simulink model "modelo_planta_CODESYS_EXPERIMENTAL"  (R2025b)
settings: Solver=FixedStepAuto  StartTime=0.0  StopTime=inf  FixedStep=Ts2  MaxStep=1e-3  RelTol=1e-3
undefined symbols (not defined in the file): ah_max, at_max, bcx, bcy, bh_eq, bhb, bhEb, bhwu, bt, bt_eq, btb, btw, g, Hc, ih, it, Jh_eq, Jt_eq, Kcy, khwu, Ki_h, Ki_t, Kp_h, Kp_t, Ktw, lambda, Lh, Lh0, lh_0, Lt, magnitude, Mc_max, Ms, Mt, rhd, rtd, tau_hm, tau_tm, Thb_Max, ThEb_Max, Thm_0, Thm_Max, titahm_0, titatm_0, Ts0, Ts1, Ts2, Ttb_Max, Ttm_0, Ttm_Max, vh_0, vlx_0, vly_0, vt_0, vt_max, Wc, whm_0, whm_rated, wtm_0, xl_0 ... (+9)
libraries: simulink x10, opcualib x9, sl3dlib x1, simulink_extras x1, dspnetwork x1
(part 1 of 2)
settings Model: SimulationMode=accelerator  Creator=Nahuel  LastModifiedBy=rodri
settings SolverCC: ZeroCrossControl=DisableAll
settings DebuggingCC: UnderSpecifiedDimensionMsg=warning
settings SFSimCC: SimTargetLang=C++  SimDLTargetLibrary=mkl-dnn
settings RTWCC: GPUComputeCapability=3.5

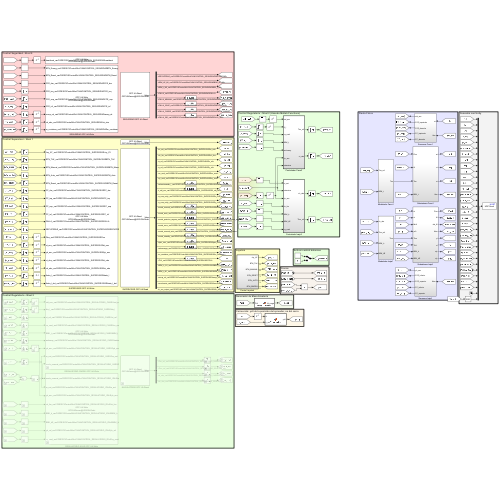
[thumbnail: Simulink's stored preview of the top-level diagram]
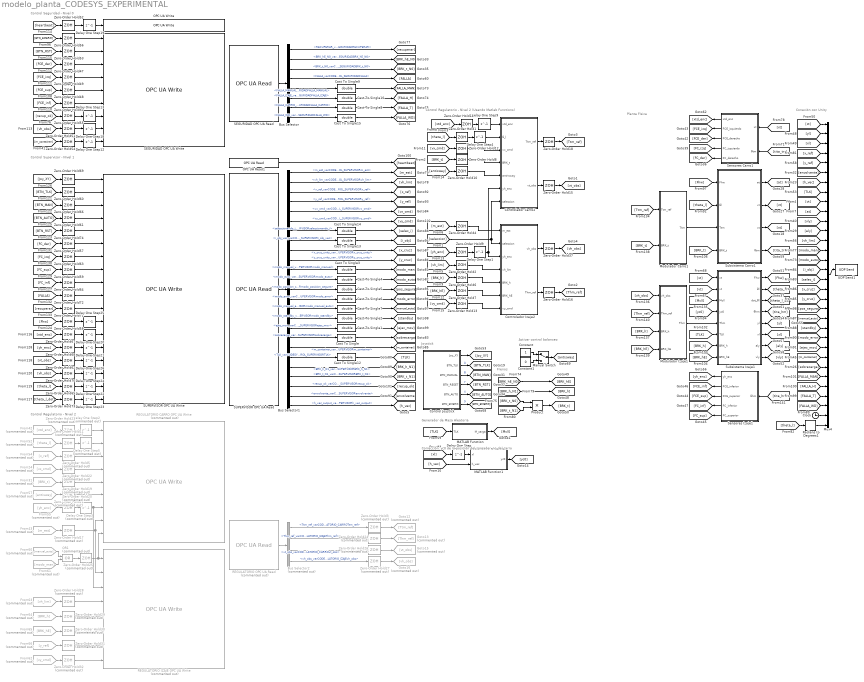
== system modelo_planta_CODESYS_EXPERIMENTAL ==
  note: Activar control balanceo
  note: Generador de Masa Aleatoria
  note: Frenos
  note: Corrección: yc0 de la posición del spreader, no del carro
  note: Joystick
  note: Conexión con Unity
  note: Control Seguridad - Nivel 0
  note: Control Supervisor - Nivel 1
  note: Control Regulatorio - Nivel 2
  note: Planta Física
  note: Control Regulatorio - Nivel 2 (Usando Matlab Functions)
  Bus Selector : BusSelector  OutputSignals=RECUPERAR_varCODESYSControlWinV3X64CONTROL_SEGURIDADRECUPERAR,BRK_hE_N0_varCODESYSControlWinV3X64CONTROL_SEGURIDADBRK_hE_N0,BRK_t_N0_varCODESYSControlWinV3X64CONTROL_SEGURIDADBRK_t_N0,FALLA_varCODESYSControlWinV3X64CONTROL_SEGURIDADFALLA,FALLA_MANUAL_varCODESYSControlWinV3X64CONTROL_SEGURIDADFALLA_MANUAL,FALLA_IZAJE_varCODESYSControlWinV3X64CONTROL_SEGURIDADFALLA_IZAJE,FALLA_CARRO_varCODESYSControlWinV3X64CONTROL_SEGURIDADFALLA_CARRO,FALLA_WD_varCODESYSControlWinV3X64CONTROL_SEGURIDADFALLA_WD
  Bus Selector1 : BusSelector  OutputSignals=m_est_varCODESYSControlWinV3X64CONTROL_SUPERVISORm_est,vh_lim_varCODESYSControlWinV3X64CONTROL_SUPERVISORvh_lim,x_ref_varCODESYSControlWinV3X64CONTROL_SUPERVISORx_ref,y_ref_varCODESYSControlWinV3X64CONTROL_SUPERVISORy_ref,vx_cmd_varCODESYSControlWinV3X64CONTROL_SUPERVISORvx_cmd,vy_cmd_varCODESYSControlWinV3X64CONTROL_SUPERVISORvy_cmd,seleccionando_i_varCODESYSControlWinV3X64CONTROL_SUPERVISORseleccionando_i,i_obj_vec_varCODESYSControlWinV3X64CONTROL_SUPERVISORi_obj_vec,x_cruz_unity_varCODESYSControlWinV3X64CONTROL_SUPERVISORx_cruz_unity,y_cruz_unity_varCODESYSControlWinV3X64CONTROL_SUPERVISORy_cruz_unity,modo_manual_varCODESYSControlWinV3X64CONTROL_SUPERVISORmodo_manual,modo_auto_varCODESYSControlWinV3X64CONTROL_SUPERVISORmodo_auto,modo_posicion_segura_varCODESYSControlWinV3X64CONTROL_SUPERVISORmodo_posicion_segura,modo_error_varCODESYSControlWinV3X64CONTROL_SUPERVISORmodo_error,modo_manual_auto_varCODESYSControlWinV3X64CONTROL_SUPERVISORmodo_manual_auto,modo_standby_varCODESYSControlWinV3X64CONTROL_SUPERVISORmodo_standby,ejec_mov_varCODESYSControlWinV3X64CONTROL_SUPERVISORejec_mov,sobrecarga_varCODESYSControlWinV3X64CONTROL_SUPERVISORsobrecarga,m_container_varCODESYSControlWinV3X64CONTROL_SUPERVISORm_container,TLK_varCODESYSControlWinV3X64CONTROL_SUPERVISORTLK,BRK_h_N1_varCODESYSControlWinV3X64CONTROL_SUPERVISORBRK_h_N1,BRK_t_N1_varCODESYSControlWinV3X64CONTROL_SUPERVISORBRK_t_N1,recup_ok_varCODESYSControlWinV3X64CONTROL_SUPERVISORrecup_ok,envolvente_varCODESYSControlWinV3X64CONTROL_SUPERVISORenvolvente,h_vec_output_varCODESYSControlWinV3X64CONTROL_SUPERVISORh_vec_output
  Bus Selector2 : BusSelector  Commented=on  OutputSignals=Ttm_ref_varCODESYSControlWinV3X64CONTROL_REGULATORIO_CARROTtm_ref,Thm_ref_varCODESYSControlWinV3X64CONTROL_REGULATORIO_IZAJEThm_ref,vt_obs_varCODESYSControlWinV3X64CONTROL_REGULATORIO_CARROvt_obs,vh_obs_varCODESYSControlWinV3X64CONTROL_REGULATORIO_IZAJEvh_obs
  Cast To Single{,1..10,12..15} (15 alike) : DataTypeConversion  OutDataTypeStr=double  SaturateOnIntegerOverflow=off  RndMeth=Floor
  Clock : Clock
  Constant : Constant
  Constant1 : Constant  Value=0
  "Control Joystick " : Subsystem  TreatAsAtomicUnit=on  SystemSampleTime=Ts2
  Controlador Carro2 : Subsystem  Priority=3  TreatAsAtomicUnit=on  SystemSampleTime=Ts2
  Controlador Izaje2 : Subsystem  Priority=3  TreatAsAtomicUnit=on  SystemSampleTime=Ts2
  Delay One Step : Delay  DelayLength=1  InitialCondition=xl_0
  Delay One Step1 : Delay  DelayLength=1  InitialCondition=yh_0
  Delay One Step{4,12..13,18..19,22..24,26} (9 alike) : Delay  DelayLength=1  InitialCondition=0
  Delay One Step2 : Delay  Commented=on  DelayLength=1  InitialCondition=xtd_0
  Delay One Step20 : Delay  DelayLength=1  InitialCondition=xt_0
  Delay One Step21 : Delay  DelayLength=1  InitialCondition=yh_0
  Delay One Step25 : Delay  DelayLength=1
  Delay One Step3 : Delay  Commented=on  DelayLength=1  InitialCondition=yh_0
  Delay One Step5 : Delay  Commented=on  DelayLength=1  InitialCondition=0
  Delay One Step9 : Delay  DelayLength=1  InitialCondition=xtd_0
  From24 : From  Commented=on  GotoTag=vx_cmd
  From31 : From  Commented=on  GotoTag=BRK_t
  From42 : From  Commented=on  GotoTag=xtd_enc
  From43 : From  Commented=on  GotoTag=m_est
  From52 : From  Commented=on  GotoTag=theta_l
  From54 : From  Commented=on  GotoTag=x_ref
  From55 : From  Commented=on  GotoTag=yh_enc
  From57 : From  Commented=on  GotoTag=antisway
  From60 : From  Commented=on  GotoTag=manual_auto
  From61 : From  Commented=on  GotoTag=modo_man
  From62 : From  Commented=on  GotoTag=vy_cmd
  From63 : From  Commented=on  GotoTag=vh_lim
  From64 : From  Commented=on  GotoTag=BRK_h
  From65 : From  Commented=on  GotoTag=BRK_hE
  From66 : From  Commented=on  GotoTag=y_ref
  Goto12 : Goto  Commented=on  GotoTag=Ttm_ref
  Goto13 : Goto  Commented=on  GotoTag=Thm_ref
  Goto15 : Goto  Commented=on  GotoTag=vt_obs
  Goto16 : Goto  Commented=on  GotoTag=vh_obs
  MATLAB Function : MATLAB Function  TreatAsAtomicUnit=on
  MATLAB Function1 : MATLAB Function  TreatAsAtomicUnit=on
  Manual Switch : ManualSwitch
  Modulador Carro1 : Subsystem
  Modulador Izaje1 : Subsystem
  Mux4 : Mux  Inputs=32
  OPC UA Read1 : opcualib/OPC UA Read  SelectedServer=OPCUAServer@LEGION-Rodri  ServerList=OPCUAServer@LEGION-Rodri  NodeList={ '1', 'heartbeat', '4', '|var|CODESYS Control Win V3 x64.CONTROL_SUPERVISOR.heartbeat', '0' }  ShowQualityPort=off  ShowTimestampPort=off  ShowTimestampPortAs=Seconds since start  SampleTime=Ts1
  OPC UA Write : opcualib/OPC UA Write  SelectedServer=OPCUAServer@LEGION-Rodri  ServerList=OPCUAServer@LEGION-Rodri  SampleTime=Ts0  NodeList={ '1', 'heartbeat', '4', '|var|CODESYS Control Win V3 x64.CONTROL_SEGURIDAD.heartbeat', '0' }
  OR1 : Logic  Commented=on  Operator=OR  IconShape=distinctive  AllPortsSameDT=off  OutDataTypeStr=boolean
  Product : Product
  REGULATORIO CARRO OPC UA Write : opcualib/OPC UA Write  Commented=on  SelectedServer=OPCUAServer@LEGION-Rodri  ServerList=OPCUAServer@LEGION-Rodri  SampleTime=0.1  NodeList={ '1', 'xtd_enc', '4', '|var|CODESYS Control Win V3 x64.CONTROL_REGULATORIO_CARRO.xtd_enc', '0'; '2', 'tita_l', '4', '|var|CODESYS Control Win V3 x64.CONTROL_REGULATORIO_CARRO.tita_l', '0'; '3', 'xt_ref', '4', '|var|CODESYS Control Win V3 x64.CONTROL_REGULATORIO_CARRO.xt_ref', '0'; '4', 'vx_cmd', '4', '|var|CODESYS Control Win V3 x64.CONTROL_REGULATORIO_CARRO.vx_cmd', '0'; '5', 'BRK_t', '4', '|var|CODESYS Control Win V3 x64.CONTROL_REGULATORIO_CARRO.BRK_t', '0'; '6', 'antisway', '4', '|var|CODESYS Control Win V3 x64.CONTROL_REGULATORIO_CARRO.antisway', '0'; '7', 'yh_enc', '4', '|var|CODESYS Control Win V3 x64.CONTROL_REGULATORIO_CARRO.yh_enc', '0'; '8', 'm_est', '4', '|var|CODESYS Control Win V3 x64.CONTROL_REGULATORIO_CARRO.m_est', '0'; '9', 'modo_manual', '4', '|var|CODESYS Control Win V3 x64.CONTROL_REGULATORIO_CARRO.modo_manual', '0' }
  REGULATORIO IZAJE OPC UA Write : opcualib/OPC UA Write  Commented=on  SelectedServer=OPCUAServer@LEGION-Rodri  ServerList=OPCUAServer@LEGION-Rodri  SampleTime=0.1  NodeList={ '1', 'modo_manual', '4', '|var|CODESYS Control Win V3 x64.CONTROL_REGULATORIO_IZAJE.modo_manual', '0'; '2', 'm_est', '4', '|var|CODESYS Control Win V3 x64.CONTROL_REGULATORIO_IZAJE.m_est', '0'; '3', 'yh_enc', '4', '|var|CODESYS Control Win V3 x64.CONTROL_REGULATORIO_IZAJE.yh_enc', '0'; '4', 'vh_lim', '4', '|var|CODESYS Control Win V3 x64.CONTROL_REGULATORIO_IZAJE.vh_lim', '0'; '5', 'BRK_h', '4', '|var|CODESYS Control Win V3 x64.CONTROL_REGULATORIO_IZAJE.BRK_h', '0'; '6', 'BRK_hE', '4', '|var|CODESYS Control Win V3 x64.CONTROL_REGULATORIO_IZAJE.BRK_hE', '0'; '7', 'yh_ref', '4', '|var|CODESYS Control Win V3 x64.CONTROL_REGULATORIO_IZAJE.yh_ref', '0'; '8', 'vy_cmd', '4', '|var|CODESYS Control Win V3 x64.CONTROL_REGULATORIO_IZAJE.vy_cmd', '0' }
  REGULATORIO OPC UA Read : opcualib/OPC UA Read  Commented=on  SelectedServer=OPCUAServer@LEGION-Rodri  ServerList=OPCUAServer@LEGION-Rodri  NodeList={ '1', 'Ttm_ref', '4', '|var|CODESYS Control Win V3 x64.CONTROL_REGULATORIO_CARRO.Ttm_ref', '0'; '2', 'Thm_ref', '4', '|var|CODESYS Control Win V3 x64.CONTROL_REGULATORIO_IZAJE.Thm_ref', '0'; '3', 'vt_obs', '4', '|var|CODESYS Control Win V3 x64.CONTROL_REGULATORIO_CARRO.vt_obs', '0'; '4', 'vh_obs', '4', '|var|CODESYS Control Win V3 x64.CONTROL_REGULATORIO_IZAJE.vh_obs', '0' }  ShowQualityPort=off  ShowTimestampPort=off  ShowTimestampPortAs=Seconds since start  SampleTime=0.1
  Radians to Degrees1 : simulink_extras/Transformations/Radians to Degrees
  SEGURIDAD OPC UA Read : opcualib/OPC UA Read  SelectedServer=OPCUAServer@LEGION-Rodri  ServerList=OPCUAServer@LEGION-Rodri  NodeList={ '1', 'RECUPERAR', '4', '|var|CODESYS Control Win V3 x64.CONTROL_SEGURIDAD.RECUPERAR', '0'; '2', 'BRK_hE_N0', '4', '|var|CODESYS Control Win V3 x64.CONTROL_SEGURIDAD.BRK_hE_N0', '0'; '3', 'BRK_t_N0', '4', '|var|CODESYS Control Win V3 x64.CONTROL_SEGURIDAD.BRK_t_N0', '0'; '4', 'FALLA', '4', '|var|CODESYS Control Win V3 x64.CONTROL_SEGURIDAD.FALLA', '0'; '5', 'FALLA_MANUAL', '4', '|var|CODESYS Control Win V3 x64.CONTROL_SEGURIDAD.FALLA_MANUAL', '0'; '6', 'FALLA_IZAJE', '4', '|var|CODESYS Control Win V3 x64.CONTROL_SEGURIDAD.FALLA_IZAJE', '0'; '7', 'FALLA_CARRO', '4', '|var|CODESYS Control Win V3 x64.CONTROL_SEGURIDAD.FALLA_CARRO', '0'; '8', 'FALLA_WD', '4', '|var|CODESYS Control Win V3 x64.CONTROL_SEGURIDAD.FALLA_WD', '0' }  ShowQualityPort=off  ShowTimestampPort=off  ShowTimestampPortAs=Seconds since start  SampleTime=0.5
  SEGURIDAD OPC UA Write : opcualib/OPC UA Write  SelectedServer=OPCUAServer@LEGION-Rodri  ServerList=OPCUAServer@LEGION-Rodri  SampleTime=0.5  NodeList={ '1', 'BTN_Emerg', '4', '|var|CODESYS Control Win V3 x64.CONTROL_SEGURIDAD.BTN_Emerg', '0'; '2', 'BTN_Reset', '4', '|var|CODESYS Control Win V3 x64.CONTROL_SEGURIDAD.BTN_Reset', '0'; '3', 'FCE_der', '4', '|var|CODESYS Control Win V3 x64.CONTROL_SEGURIDAD.FCE_der', '0'; '4', 'FCE_izq', '4', '|var|CODESYS Control Win V3 x64.CONTROL_SEGURIDAD.FCE_izq', '0'; '5', 'FCE_sup', '4', '|var|CODESYS Control Win V3 x64.CONTROL_SEGURIDAD.FCE_sup', '0'; '6', 'FCE_inf', '4', '|var|CODESYS Control Win V3 x64.CONTROL_SEGURIDAD.FCE_inf', '0'; '7', 'recup_ok', '4', '|var|CODESYS Control Win V3 x64.CONTROL_SEGURIDAD.recup_ok', '0'; '8', 'vh_obs', '4', '|var|CODESYS Control Win V3 x64.CONTROL_SEGURIDAD.vh_obs', '0'; '9', 'm_container', '4', '|var|CODESYS Control Win V3 x64.CONTROL_SEGURIDAD.m_container', '0' }
  SUPERVISOR OPC UA Read : opcualib/OPC UA Read  SelectedServer=OPCUAServer@LEGION-Rodri  ServerList=OPCUAServer@LEGION-Rodri  NodeList={ '1', 'm_est', '4', '|var|CODESYS Control Win V3 x64.CONTROL_SUPERVISOR.m_est', '0'; '2', 'vh_lim', '4', '|var|CODESYS Control Win V3 x64.CONTROL_SUPERVISOR.vh_lim', '0'; '3', 'x_ref', '4', '|var|CODESYS Control Win V3 x64.CONTROL_SUPERVISOR.x_ref', '0'; '4', 'y_ref', '4', '|var|CODESYS Control Win V3 x64.CONTROL_SUPERVISOR.y_ref', '0'; '5', 'vx_cmd', '4', '|var|CODESYS Control Win V3 x64.CONTROL_SUPERVISOR.vx_cmd', '0'; '6', 'vy_cmd', '4', '|var|CODESYS Control Win V3 x64.CONTROL_SUPERVISOR.vy_cmd', '0'; '7', 'seleccionando_i', '4', '|var|CODESYS Control Win V3 x64.CONTROL_SUPERVISOR.seleccionando_i', '0'; '8', 'i_obj_vec', '4', '|var|CODESYS Control Win V3 x64.CONTROL_SUPERVISOR.i_obj_vec', '0'; '9', 'x_cruz_unity', '4', '|var|CODESYS Control Win V3 x64.CONTROL_SUPERVISOR.x_cruz_unity', '0'; '10', 'y_cruz_unity', '4', '|var|CODESYS Control Win V3 x64.CONTROL_SUPERVISOR.y_cruz_unity', '0'; '11', 'modo_manual', '4', '|var|CODESYS Control Win V3 x64.CONTROL_SUPERVISOR.modo_manual', '0'; '12', 'modo_auto', '4', '|var|CODESYS Control Win V3 x64.CONTROL_SUPERVISOR.modo_auto', '0'; '13', 'modo_posicion_segura', '4', '|var|CODESYS Control Win V3 x64.CONTROL_SUPERVISOR.modo_posicion_segura', '0'; '14', 'modo_error', '4', '|var|CODESYS Control Win V3 x64.CONTROL_SUPERVISOR.modo_error', '0'; '15', 'modo_manual_auto', '4', '|var|CODESYS Control Win V3 x64.CONTROL_SUPERVISOR.modo_manual_auto', '0'; '16', 'modo_standby', '4', '|var|CODESYS Control Win V3 x64.CONTROL_SUPERVISOR.modo_standby', '0'; '17', 'ejec_mov', '4', '|var|CODESYS Control Win V3 x64.CONTROL_SUPERVISOR.ejec_mov', '0'; '18', 'sobrecarga', '4', '|var|CODESYS Control Win V3 x64.CONTROL_SUPERVISOR.sobrecarga', '0'; '19', 'm_container', '4', '|var|CODESYS Control Win V3 x64.CONTROL_SUPERVISOR.m_container', '0'; '20', 'TLK', '4', '|var|CODESYS Control Win V3 x64.CONTROL_SUPERVISOR.TLK', '0'; '21', 'BRK_h_N1', '4', '|var|CODESYS Control Win V3 x64.CONTROL_SUPERVISOR.BRK_h_N1', '0'; '22', 'BRK_t_N1', '4', '|var|CODESYS Control Win V3 x64.CONTROL_SUPERVISOR.BRK_t_N1', '0'; '23', 'recup_ok', '4', '|var|CODESYS Control Win V3 x64.CONTROL_SUPERVISOR.recup_ok', '0'; '24', 'envolvente', '4', '|var|CODESYS Control Win V3 x64.CONTROL_SUPERVISOR.envolvente', '0'; '25', 'h_vec_output', '4', '|var|CODESYS Control Win V3 x64.CONTROL_SUPERVISOR.h_vec_output', '0' }  ShowQualityPort=off  ShowTimestampPort=off  ShowTimestampPortAs=Seconds since start  SampleTime=0.5
  SUPERVISOR OPC UA Write : opcualib/OPC UA Write  SelectedServer=OPCUAServer@LEGION-Rodri  ServerList=OPCUAServer@LEGION-Rodri  SampleTime=0.5  NodeList={ '1', 'Joy_XY', '4', '|var|CODESYS Control Win V3 x64.CONTROL_SUPERVISOR.Joy_XY', '0'; '2', 'BTN_TLK', '4', '|var|CODESYS Control Win V3 x64.CONTROL_SUPERVISOR.BTN_TLK', '0'; '3', 'BTN_Manual', '4', '|var|CODESYS Control Win V3 x64.CONTROL_SUPERVISOR.BTN_Manual', '0'; '4', 'BTN_Auto', '4', '|var|CODESYS Control Win V3 x64.CONTROL_SUPERVISOR.BTN_Auto', '0'; '5', 'BTN_Reset', '4', '|var|CODESYS Control Win V3 x64.CONTROL_SUPERVISOR.BTN_Reset', '0'; '6', 'FC_der', '4', '|var|CODESYS Control Win V3 x64.CONTROL_SUPERVISOR.FC_der', '0'; '7', 'FC_izq', '4', '|var|CODESYS Control Win V3 x64.CONTROL_SUPERVISOR.FC_izq', '0'; '8', 'FC_sup', '4', '|var|CODESYS Control Win V3 x64.CONTROL_SUPERVISOR.FC_sup', '0'; '9', 'FC_inf', '4', '|var|CODESYS Control Win V3 x64.CONTROL_SUPERVISOR.FC_inf', '0'; '10', 'FALLA', '4', '|var|CODESYS Control Win V3 x64.CONTROL_SUPERVISOR.FALLA', '0'; '11', 'RECUPERAR', '4', '|var|CODESYS Control Win V3 x64.CONTROL_SUPERVISOR.RECUPERAR', '0'; '12', 'Fhw', '4', '|var|CODESYS Control Win V3 x64.CONTROL_SUPERVISOR.Fhw', '0'; '13', 'xt_enc', '4', '|var|CODESYS Control Win V3 x64.CONTROL_SUPERVISOR.xt_enc', '0'; '14', 'yh_enc', '4', '|var|CODESYS Control Win V3 x64.CONTROL_SUPERVISOR.yh_enc', '0'; '15', 'vt_obs', '4', '|var|CODESYS Control Win V3 x64.CONTROL_SUPERVISOR.vt_obs', '0'; '16', 'vh_obs', '4', '|var|CODESYS Control Win V3 x64.CONTROL_SUPERVISOR.vh_obs', '0'; '17', 'theta_l', '4', '|var|CODESYS Control Win V3 x64.CONTROL_SUPERVISOR.theta_l', '0'; '18', 'theta_l_dot', '4', '|var|CODESYS Control Win V3 x64.CONTROL_SUPERVISOR.theta_l_dot', '0' }
  Sensores Carro1 : Subsystem
  Sensores Izaje1 : Subsystem
  Subsistema Carro1 : Subsystem
  Subsistema Izaje1 : Subsystem
  UDP Send1 : dspnetwork/UDP Send  remoteURL='127.0.0.1'  remotePort=1234  localURL='0.0.0.0'  localPortSource=Automatically determine  localPort=-1  sendBufferSize=8192  sampletime=-1  blockPlatform=HOST  separateLengthPort=0
  Zero-Order Hold{1..2,4,6..10,12..16,18,37} (15 alike) : ZeroOrderHold  SampleTime=Ts2
  Zero-Order Hold{3,5,11,17,19..32} (18 alike) : ZeroOrderHold  Commented=on  SampleTime=Ts2
  Zero-Order Hold{47..56} (10 alike) : ZeroOrderHold  SampleTime=Ts0
  Zero-Order Hold{57..74} (18 alike) : ZeroOrderHold  SampleTime=Ts1
  wires:
  [BRK_t_N0] -> Product/1
  [BRK_t_N1] -> Product/2
  [BRK_h_N1] -> [BRK_h]
  [BRK_hE_N0] -> [BRK_hE]
  Product/1 -> [BRK_t]
  "Control Joystick "/2(BTN_TLK) -> [BTN_TLK]  "A"
  "Control Joystick "/1(Joy_XY) -> [Joy_XY]
  "Control Joystick "/5(BTN_AUTO) -> [BTN_AUTO]  "X"
  "Control Joystick "/4(BTN_RESET) -> [BTN_RST]  "Y"
  "Control Joystick "/3(BTN_MANUAL) -> [BTN_MAN]  "B"
  [TLK] -> MATLAB Function/1(TLK)
  MATLAB Function/1(M_carga) -> [McX]
  [vh_lim] -> Mux4/13
  [at] -> Mux4/10
  [vt] -> Mux4/9
  [xt] -> Mux4/1
  [envolvente] -> Mux4/6
  [vly] -> Mux4/11
  [h_vec] -> Mux4/7
  [yl] -> Mux4/2
  [y_ref] -> Mux4/5
  [TLK] -> Mux4/8
  [xl] -> Mux4/3
  [x_ref] -> Mux4/4
  Mux4/1 -> UDP Send1/1
  [modo_man] -> Mux4/14
  [modo_auto] -> Mux4/15
  [i_obj] -> Mux4/16
  [selec_i] -> Mux4/17
  [x_cruz] -> Mux4/18
  [y_cruz] -> Mux4/19
  [pos_segura] -> Mux4/20
  [manual_auto] -> Mux4/21
  [standby] -> Mux4/22
  [modo_error] -> Mux4/23
  [ejec_mov] -> Mux4/24
  [m_container] -> Mux4/25
  [sobrecarga] -> Mux4/26
  MATLAB Function1/1(yc0) -> [yc0]
  [xl] -> Delay One Step/1
  Delay One Step/1 -> MATLAB Function1/1(xl)
  [h_vec] -> MATLAB Function1/2(h_vec)
  [aly] -> Mux4/12
  [FALLA_MAN] -> Mux4/27
  [FALLA_H] -> Mux4/28
  [FALLA_T] -> Mux4/29
  [FALLA_WD] -> Mux4/30
  "Control Joystick "/6(BTN_EMERG) -> [BTN_EMERG]  "9"
  Constant/1 -> Manual Switch/1
  Manual Switch/1 -> [antisway]
  Constant1/1 -> Manual Switch/2
  SEGURIDAD OPC UA Read/1 -> Bus Selector/1
  Zero-Order Hold55/1 -> Delay One Step13/1
  [FCE_inf] -> Zero-Order Hold50/1
  [FCE_der] -> Zero-Order Hold47/1
  [m_container] -> Zero-Order Hold54/1
  Zero-Order Hold54/1 -> Delay One Step12/1
  [BTN_RST] -> Zero-Order Hold53/1
  [vh_obs] -> Zero-Order Hold51/1
  [FCE_izq] -> Zero-Order Hold49/1
  Zero-Order Hold51/1 -> Delay One Step18/1
  [recup_ok] -> Zero-Order Hold55/1
  [BTN_EMERG] -> Zero-Order Hold56/1
  [FCE_sup] -> Zero-Order Hold48/1
  Delay One Step12/1 -> SEGURIDAD OPC UA Write/9
  Delay One Step18/1 -> SEGURIDAD OPC UA Write/8
  Bus Selector/1 -> [recuperar]  "<RECUPERAR_varCODESYSControlWinV3X64CONTROL_SEGURIDADRECUPERAR>"
  Bus Selector/2 -> [BRK_hE_N0]  "<BRK_hE_N0_varCODESYSControlWinV3X64CONTROL_SEGURIDADBRK_hE_N0>"
  Bus Selector/3 -> [BRK_t_N0]  "<BRK_t_N0_varCODESYSControlWinV3X64CONTROL_SEGURIDADBRK_t_N0>"
  Bus Selector/4 -> [FALLA]  "<FALLA_varCODESYSControlWinV3X64CONTROL_SEGURIDADFALLA>"
  Bus Selector/5 -> Cast To Single9/1  "<FALLA_MANUAL_varCODESYSControlWinV3X64CONTROL_SEGURIDADFALLA_MANUAL>"
  Bus Selector/6 -> Cast To Single10/1  "<FALLA_IZAJE_varCODESYSControlWinV3X64CONTROL_SEGURIDADFALLA_IZAJE>"
  Bus Selector/7 -> Cast To Single8/1  "<FALLA_CARRO_varCODESYSControlWinV3X64CONTROL_SEGURIDADFALLA_CARRO>"
  Bus Selector/8 -> Cast To Single15/1  "<FALLA_WD_varCODESYSControlWinV3X64CONTROL_SEGURIDADFALLA_WD>"
  Zero-Order Hold56/1 -> SEGURIDAD OPC UA Write/1
  Zero-Order Hold53/1 -> SEGURIDAD OPC UA Write/2
  Zero-Order Hold47/1 -> SEGURIDAD OPC UA Write/3
  Zero-Order Hold49/1 -> SEGURIDAD OPC UA Write/4
  Zero-Order Hold48/1 -> SEGURIDAD OPC UA Write/5
  Zero-Order Hold50/1 -> SEGURIDAD OPC UA Write/6
  Delay One Step13/1 -> SEGURIDAD OPC UA Write/7
  Cast To Single8/1 -> [FALLA_T]
  Cast To Single10/1 -> [FALLA_H]
  Cast To Single9/1 -> [FALLA_MAN]
  [yh_enc] -> Zero-Order Hold68/1
  [vh_obs] -> Zero-Order Hold70/1
  [FC_izq] -> Zero-Order Hold63/1
  [theta_l_dot] -> Zero-Order Hold73/1
  Zero-Order Hold68/1 -> Delay One Step21/1
  [FALLA] -> Zero-Order Hold72/1
  [BTN_MAN] -> Zero-Order Hold66/1
  [FC_der] -> Zero-Order Hold57/1
  Zero-Order Hold73/1 -> Delay One Step23/1
  Zero-Order Hold65/1 -> Delay One Step22/1
  [FC_inf] -> Zero-Order Hold64/1
  [BTN_TLK] -> Zero-Order Hold60/1
  Zero-Order Hold62/1 -> Delay One Step26/1
  [Fhw] -> Zero-Order Hold58/1
  [BTN_AUTO] -> Zero-Order Hold61/1
  [theta_l] -> Zero-Order Hold65/1
  [xtd_enc] -> Zero-Order Hold67/1
  [BTN_RST] -> Zero-Order Hold74/1
  [FC_sup] -> Zero-Order Hold59/1
  Zero-Order Hold70/1 -> Delay One Step24/1
  Zero-Order Hold58/1 -> Delay One Step25/1
  Zero-Order Hold67/1 -> Delay One Step20/1
  [recuperar] -> Zero-Order Hold71/1
  [vt_obs] -> Zero-Order Hold62/1
  Zero-Order Hold66/1 -> SUPERVISOR OPC UA Write/3
  Zero-Order Hold61/1 -> SUPERVISOR OPC UA Write/4
  Zero-Order Hold74/1 -> SUPERVISOR OPC UA Write/5
  Zero-Order Hold57/1 -> SUPERVISOR OPC UA Write/6
  Zero-Order Hold63/1 -> SUPERVISOR OPC UA Write/7
  Zero-Order Hold59/1 -> SUPERVISOR OPC UA Write/8
  Zero-Order Hold64/1 -> SUPERVISOR OPC UA Write/9
  Zero-Order Hold72/1 -> SUPERVISOR OPC UA Write/10
  Zero-Order Hold71/1 -> SUPERVISOR OPC UA Write/11
  Zero-Order Hold60/1 -> SUPERVISOR OPC UA Write/2
  Delay One Step25/1 -> SUPERVISOR OPC UA Write/12
  Delay One Step20/1 -> SUPERVISOR OPC UA Write/13
  Delay One Step21/1 -> SUPERVISOR OPC UA Write/14
  Delay One Step26/1 -> SUPERVISOR OPC UA Write/15
  Delay One Step24/1 -> SUPERVISOR OPC UA Write/16
  Delay One Step22/1 -> SUPERVISOR OPC UA Write/17
  Delay One Step23/1 -> SUPERVISOR OPC UA Write/18
  Bus Selector1/1 -> [m_est]  "<m_est_varCODESYSControlWinV3X64CONTROL_SUPERVISORm_est>"
  Bus Selector1/2 -> [vh_lim]  "<vh_lim_varCODESYSControlWinV3X64CONTROL_SUPERVISORvh_lim>"
  Bus Selector1/3 -> [x_ref]  "<x_ref_varCODESYSControlWinV3X64CONTROL_SUPERVISORx_ref>"
  Bus Selector1/4 -> [y_ref]  "<y_ref_varCODESYSControlWinV3X64CONTROL_SUPERVISORy_ref>"
  Bus Selector1/5 -> [vx_cmd]  "<vx_cmd_varCODESYSControlWinV3X64CONTROL_SUPERVISORvx_cmd>"
  Bus Selector1/6 -> [vy_cmd]  "<vy_cmd_varCODESYSControlWinV3X64CONTROL_SUPERVISORvy_cmd>"
  Bus Selector1/7 -> Cast To Single14/1  "<seleccionando_i_varCODESYSControlWinV3X64CONTROL_SUPERVISORseleccionando_i>"
  Bus Selector1/8 -> Cast To Single13/1  "<i_obj_vec_varCODESYSControlWinV3X64CONTROL_SUPERVISORi_obj_vec>"
  Bus Selector1/9 -> [x_cruz]  "<x_cruz_unity_varCODESYSControlWinV3X64CONTROL_SUPERVISORx_cruz_unity>"
  Bus Selector1/10 -> [y_cruz]  "<y_cruz_unity_varCODESYSControlWinV3X64CONTROL_SUPERVISORy_cruz_unity>"
  Bus Selector1/11 -> Cast To Single3/1  "<modo_manual_varCODESYSControlWinV3X64CONTROL_SUPERVISORmodo_manual>"
  Bus Selector1/12 -> Cast To Single4/1  "<modo_auto_varCODESYSControlWinV3X64CONTROL_SUPERVISORmodo_auto>"
  Bus Selector1/13 -> Cast To Single5/1  "<modo_posicion_segura_varCODESYSControlWinV3X64CONTROL_SUPERVISORmodo_posicion_segura>"
  Bus Selector1/14 -> Cast To Single6/1  "<modo_error_varCODESYSControlWinV3X64CONTROL_SUPERVISORmodo_error>"
  Bus Selector1/15 -> Cast To Single7/1  "<modo_manual_auto_varCODESYSControlWinV3X64CONTROL_SUPERVISORmodo_manual_auto>"
  Bus Selector1/16 -> Cast To Single2/1  "<modo_standby_varCODESYSControlWinV3X64CONTROL_SUPERVISORmodo_standby>"
  Bus Selector1/17 -> Cast To Single1/1  "<ejec_mov_varCODESYSControlWinV3X64CONTROL_SUPERVISORejec_mov>"
  Bus Selector1/18 -> Cast To Single/1  "<sobrecarga_varCODESYSControlWinV3X64CONTROL_SUPERVISORsobrecarga>"
  Bus Selector1/19 -> [m_container]  "<m_container_varCODESYSControlWinV3X64CONTROL_SUPERVISORm_container>"
  Bus Selector1/20 -> Cast To Single12/1  "<TLK_varCODESYSControlWinV3X64CONTROL_SUPERVISORTLK>"
  Bus Selector1/21 -> [BRK_h_N1]  "<BRK_h_N1_varCODESYSControlWinV3X64CONTROL_SUPERVISORBRK_h_N1>"
  Bus Selector1/22 -> [BRK_t_N1]  "<BRK_t_N1_varCODESYSControlWinV3X64CONTROL_SUPERVISORBRK_t_N1>"
  Bus Selector1/23 -> [recup_ok]  "<recup_ok_varCODESYSControlWinV3X64CONTROL_SUPERVISORrecup_ok>"
  Bus Selector1/24 -> [envolvente]  "<envolvente_varCODESYSControlWinV3X64CONTROL_SUPERVISORenvolvente>"
  Bus Selector1/25 -> [h_vec]  "<h_vec_output_varCODESYSControlWinV3X64CONTROL_SUPERVISORh_vec_output>"
  SUPERVISOR OPC UA Read/1 -> Bus Selector1/1
  Cast To Single3/1 -> [modo_man]
  Cast To Single4/1 -> [modo_auto]
  Cast To Single5/1 -> [pos_segura]
  Cast To Single6/1 -> [modo_error]
  Cast To Single7/1 -> [manual_auto]
  Cast To Single2/1 -> [standby]
  Cast To Single1/1 -> [ejec_mov]
  Cast To Single/1 -> [sobrecarga]
  Cast To Single15/1 -> [FALLA_WD]
  Cast To Single12/1 -> [TLK]
  Cast To Single13/1 -> [i_obj]
  Cast To Single14/1 -> [selec_i]
  OPC UA Read1/1 -> [heartbeat]
  [heartbeat] -> Zero-Order Hold52/1
  Zero-Order Hold52/1 -> Delay One Step19/1
  Delay One Step19/1 -> OPC UA Write/1
  [Joy_XY] -> Zero-Order Hold69/1
  Zero-Order Hold69/1 -> SUPERVISOR OPC UA Write/1
  REGULATORIO OPC UA Read/1 -> Bus Selector2/1
  Zero-Order Hold3/1 -> Goto12/1
  Zero-Order Hold5/1 -> REGULATORIO CARRO OPC UA Write/3
  From55/1 -> Zero-Order Hold20/1
  Zero-Order Hold22/1 -> REGULATORIO CARRO OPC UA Write/4
  From52/1 -> Zero-Order Hold11/1
  From54/1 -> Zero-Order Hold5/1
  Zero-Order Hold20/1 -> Delay One Step3/1
  From31/1 -> Zero-Order Hold19/1
  From24/1 -> Zero-Order Hold22/1
  Zero-Order Hold19/1 -> REGULATORIO CARRO OPC UA Write/5
  Zero-Order Hold21/1 -> REGULATORIO CARRO OPC UA Write/6
  From57/1 -> Zero-Order Hold21/1
  Zero-Order Hold11/1 -> Delay One Step5/1
  From42/1 -> Zero-Order Hold23/1
  Zero-Order Hold23/1 -> Delay One Step2/1
  From43/1 -> Zero-Order Hold17/1
  Zero-Order Hold24/1 -> Goto13/1
  OR1/1 -> Zero-Order Hold25/1
  From60/1 -> OR1/1
  From61/1 -> OR1/2
  Delay One Step2/1 -> REGULATORIO CARRO OPC UA Write/1
  Delay One Step5/1 -> REGULATORIO CARRO OPC UA Write/2
  Delay One Step3/1 -> REGULATORIO IZAJE OPC UA Write/3, REGULATORIO CARRO OPC UA Write/7
  Zero-Order Hold17/1 -> REGULATORIO IZAJE OPC UA Write/2, REGULATORIO CARRO OPC UA Write/8
  Zero-Order Hold25/1 -> REGULATORIO CARRO OPC UA Write/9, REGULATORIO IZAJE OPC UA Write/1
  Bus Selector2/1 -> Zero-Order Hold3/1  "<Ttm_ref_varCODESYSControlWinV3X64CONTROL_REGULATORIO_CARROTtm_ref>"
  Bus Selector2/2 -> Zero-Order Hold24/1  "<Thm_ref_varCODESYSControlWinV3X64CONTROL_REGULATORIO_IZAJEThm_ref>"
  Zero-Order Hold26/1 -> Goto15/1
  Bus Selector2/3 -> Zero-Order Hold26/1  "<vt_obs_varCODESYSControlWinV3X64CONTROL_REGULATORIO_CARROvt_obs>"
  Zero-Order Hold27/1 -> Goto16/1
  Bus Selector2/4 -> Zero-Order Hold27/1  "<vh_obs_varCODESYSControlWinV3X64CONTROL_REGULATORIO_IZAJEvh_obs>"
  From62/1 -> Zero-Order Hold32/1
  From63/1 -> Zero-Order Hold28/1
  From65/1 -> Zero-Order Hold30/1
  From64/1 -> Zero-Order Hold29/1
  From66/1 -> Zero-Order Hold31/1
  Zero-Order Hold32/1 -> REGULATORIO IZAJE OPC UA Write/8
  Zero-Order Hold31/1 -> REGULATORIO IZAJE OPC UA Write/7
  Zero-Order Hold30/1 -> REGULATORIO IZAJE OPC UA Write/6
  Zero-Order Hold29/1 -> REGULATORIO IZAJE OPC UA Write/5
  Zero-Order Hold28/1 -> REGULATORIO IZAJE OPC UA Write/4
  Subsistema Izaje1/8(vly) -> [vly]
  [tita_hm] -> Sensores Izaje1/1(θhm)
  Modulador Carro1/1(Ttm) -> Subsistema Carro1/3(Ttm)
  Subsistema Izaje1/5(yl) -> [yl]
  [yc0] -> Subsistema Izaje1/4(yc0)
  Sensores Carro1/3(FCE_derecho) -> [FCE_der]
  Modulador Izaje1/1(Thm) -> Subsistema Izaje1/5(Thm)
  [BRK_hE] -> Subsistema Izaje1/8(BRK_hE)
  Sensores Carro1/5(FC_derecho) -> [FC_der]
  Sensores Izaje1/3(FCE_superior) -> [FCE_sup]
  Sensores Izaje1/2(FCE_inferior) -> [FCE_inf]
  [BRK_h] -> Modulador Izaje1/3(BRK_h)
  Sensores Carro1/2(FCE_izquierdo) -> [FCE_izq]
  [tita_tm] -> Sensores Carro1/2(θtm)
  Sensores Izaje1/5(FC_superior) -> [FC_sup]
  Sensores Carro1/4(FC_izquierdo) -> [FC_izq]
  Subsistema Carro1/3(xt) -> [xt]
  [theta_l] -> Subsistema Carro1/2(θl)
  [xt] -> Subsistema Izaje1/1(xt)
  Subsistema Izaje1/6(xl) -> [xl]
  Subsistema Carro1/2(vt) -> [vt]
  [BRK_h] -> Subsistema Izaje1/7(BRK_h)
  [TLK] -> Subsistema Izaje1/6(TLK)
  [vh_obs] -> Modulador Izaje1/1(vh_obs)
  [Thm_ref] -> Modulador Izaje1/2(Thm_ref)
  Sensores Izaje1/1(yh_enc) -> [yh_enc]
  Sensores Carro1/1(xtd_enc) -> [xtd_enc]
  Subsistema Izaje1/7(aly) -> [aly]
  [vt] -> Subsistema Izaje1/2(vt)
  Subsistema Izaje1/4(θhm) -> [tita_hm]
  Subsistema Carro1/1(at) -> [at]
  [BRK_hE] -> Modulador Izaje1/4(BRK_hE)
  Sensores Izaje1/4(FC_inferior) -> [FC_inf]
  Subsistema Izaje1/2(θl) -> [theta_l]
  Subsistema Carro1/4(θtm) -> [tita_tm]
  [McX] -> Subsistema Izaje1/3(McX)
  [Ttm_ref] -> Modulador Carro1/1(Ttm_ref)
  [Fhw] -> Subsistema Carro1/1(Fhw)
  [xt] -> Sensores Carro1/1(xt)
  Subsistema Izaje1/1(Fhw) -> [Fhw]
  [BRK_t] -> Subsistema Carro1/4(BRK_t)
  Subsistema Izaje1/3(dot_θl) -> [theta_l_dot]
  [BRK_t] -> Modulador Carro1/2(BRK_t)
  Clock/1 -> Mux4/31
  [theta_l] -> Radians to Degrees1/1
  Radians to Degrees1/1 -> Mux4/32
  Zero-Order Hold13/1 -> Controlador Izaje2/7(vy_cmd)
  Controlador Izaje2/2(Thm_ref) -> Zero-Order Hold16/1
  [BRK_hE] -> Zero-Order Hold7/1
  Zero-Order Hold14/1 -> Delay One Step9/1
  [vh_lim] -> Zero-Order Hold2/1
  Zero-Order Hold18/1 -> [Ttm_ref]
  Zero-Order Hold6/1 -> Controlador Izaje2/5(BRK_h)
  [BRK_t] -> Zero-Order Hold8/1
  Zero-Order Hold1/1 -> Delay One Step4/1
  Zero-Order Hold9/1 -> Delay One Step1/1
  [xtd_enc] -> Zero-Order Hold14/1
  Zero-Order Hold37/1 -> [vh_obs]
  Zero-Order Hold16/1 -> [Thm_ref]
  Delay One Step4/1 -> Controlador Carro2/2(θ_l)
  [theta_l] -> Zero-Order Hold1/1
  [yh_enc] -> Zero-Order Hold9/1
  Zero-Order Hold2/1 -> Controlador Izaje2/4(vh_lim)
  [seleccion] -> Controlador Izaje2/2(seleccion), Controlador Carro2/7(seleccion)
  Controlador Izaje2/1(vh_obs) -> Zero-Order Hold37/1
  [m_est] -> Zero-Order Hold4/1
  [vx_cmd] -> Zero-Order Hold12/1
  [BRK_h] -> Zero-Order Hold6/1
  Zero-Order Hold4/1 -> Controlador Izaje2/1(m_est)
  Zero-Order Hold7/1 -> Controlador Izaje2/6(BRK_hE)
  Zero-Order Hold8/1 -> Controlador Carro2/4(BRK_t)
  Delay One Step9/1 -> Controlador Carro2/1(xtd_enc)
  Delay One Step1/1 -> Controlador Izaje2/3(yh_enc), Controlador Carro2/6(yh_enc)
  Controlador Carro2/2(vt_obs) -> Zero-Order Hold15/1
  Zero-Order Hold15/1 -> [vt_obs]
  Zero-Order Hold12/1 -> Controlador Carro2/3(vx_cmd)
  Controlador Carro2/1(Ttm_ref) -> Zero-Order Hold18/1
  [antisway] -> Zero-Order Hold10/1
  Zero-Order Hold10/1 -> Controlador Carro2/5(anti-sway)
  [vy_cmd] -> Zero-Order Hold13/1

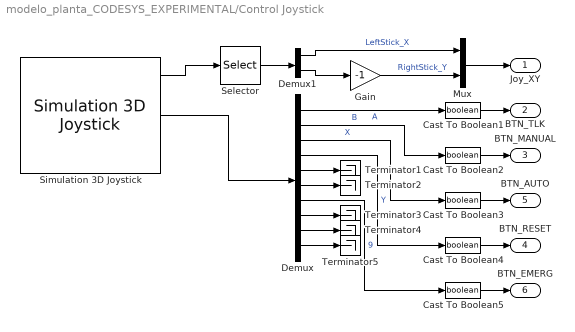
== system modelo_planta_CODESYS_EXPERIMENTAL/Control Joystick  ==
  Cast To Boolean{1..5} (5 alike) : DataTypeConversion  OutDataTypeStr=boolean  SaturateOnIntegerOverflow=off  RndMeth=Floor
  Demux : Demux  Outputs=10
  Demux1 : Demux  Outputs=2
  Gain : Gain  Gain=-1
  Mux : Mux  Inputs=2
  Selector : Selector  InputPortWidth=5  IndexOptions=Index vector (dialog)  Indices=[1 5]  OutputSizes=1
  Simulation 3D Joystick : sl3dlib/Simulation 3D/Hardware Interface/Simulation 3D Joystick  joyid=1  adjustports=on  forcefeed=off
  Terminator{1..5} (5 alike) : Terminator
  Joy_XY : Outport
  BTN_TLK : Outport  Port=2
  BTN_MANUAL : Outport  Port=3
  BTN_RESET : Outport  Port=4
  BTN_AUTO : Outport  Port=5
  BTN_EMERG : Outport  Port=6
  wires:
  Demux/1 -> Cast To Boolean1/1  "A"
  Demux1/2 -> Gain/1
  Demux1/1 -> Mux/1  "LeftStick_X"
  Selector/1 -> Demux1/1
  Simulation 3D Joystick/1 -> Selector/1
  Gain/1 -> Mux/2  "RightStick_Y"
  Simulation 3D Joystick/2 -> Demux/1
  Demux/2 -> Cast To Boolean2/1  "B"
  Demux/3 -> Cast To Boolean3/1  "X"
  Demux/4 -> Cast To Boolean4/1  "Y"
  Mux/1 -> Joy_XY/1
  Demux/5 -> Terminator1/1
  Demux/6 -> Terminator2/1
  Demux/8 -> Terminator3/1
  Demux/9 -> Terminator4/1
  Demux/10 -> Terminator5/1
  Demux/7 -> Cast To Boolean5/1  "9"
  Cast To Boolean1/1 -> BTN_TLK/1
  Cast To Boolean2/1 -> BTN_MANUAL/1
  Cast To Boolean3/1 -> BTN_AUTO/1
  Cast To Boolean4/1 -> BTN_RESET/1
  Cast To Boolean5/1 -> BTN_EMERG/1

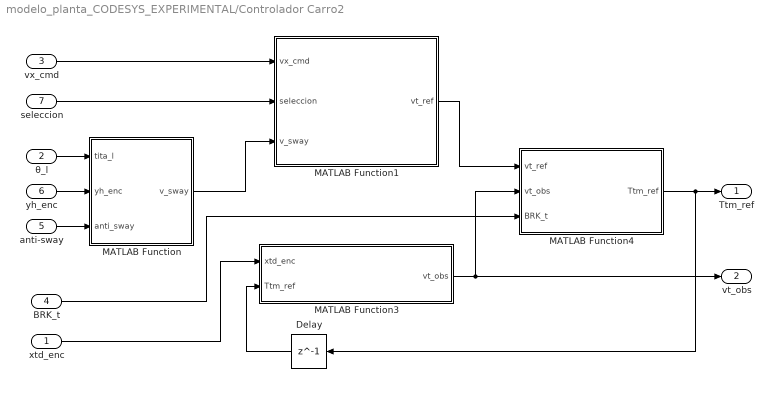
== system modelo_planta_CODESYS_EXPERIMENTAL/Controlador Carro2 ==
  xtd_enc : Inport
  θ_l : Inport  Port=2
  vx_cmd : Inport  Port=3
  BRK_t : Inport  Port=4
  anti-sway : Inport  Port=5
  yh_enc : Inport  Port=6
  seleccion : Inport  Port=7
  Delay : Delay  DelayLength=1  InitialCondition=Ttm_0
  MATLAB Function : MATLAB Function  TreatAsAtomicUnit=on
  MATLAB Function1 : MATLAB Function  TreatAsAtomicUnit=on
  MATLAB Function3 : MATLAB Function  TreatAsAtomicUnit=on
  MATLAB Function4 : MATLAB Function  TreatAsAtomicUnit=on
  Ttm_ref : Outport
  vt_obs : Outport  Port=2
  wires:
  seleccion/1 -> MATLAB Function1/2(seleccion)
  θ_l/1 -> MATLAB Function/1(tita_l)
  vx_cmd/1 -> MATLAB Function1/1(vx_cmd)
  yh_enc/1 -> MATLAB Function/2(yh_enc)
  MATLAB Function/1(v_sway) -> MATLAB Function1/3(v_sway)
  MATLAB Function3/1(vt_obs) -> vt_obs/1, MATLAB Function4/2(vt_obs)
  BRK_t/1 -> MATLAB Function4/3(BRK_t)
  Delay/1 -> MATLAB Function3/2(Ttm_ref)
  xtd_enc/1 -> MATLAB Function3/1(xtd_enc)
  MATLAB Function1/1(vt_ref) -> MATLAB Function4/1(vt_ref)
  anti-sway/1 -> MATLAB Function/3(anti_sway)
  MATLAB Function4/1(Ttm_ref) -> Ttm_ref/1, Delay/1

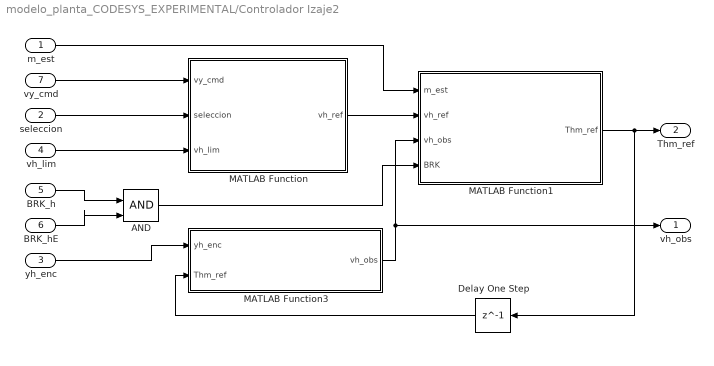
== system modelo_planta_CODESYS_EXPERIMENTAL/Controlador Izaje2 ==
  m_est : Inport
  seleccion : Inport  Port=2
  yh_enc : Inport  Port=3
  vh_lim : Inport  Port=4
  BRK_h : Inport  Port=5
  BRK_hE : Inport  Port=6
  vy_cmd : Inport  Port=7
  AND : Logic  IconShape=distinctive  AllPortsSameDT=off  OutDataTypeStr=boolean
  Delay One Step : Delay  DelayLength=1  InitialCondition=Thm_0
  MATLAB Function : MATLAB Function  TreatAsAtomicUnit=on
  MATLAB Function1 : MATLAB Function  TreatAsAtomicUnit=on
  MATLAB Function3 : MATLAB Function  TreatAsAtomicUnit=on
  vh_obs : Outport
  Thm_ref : Outport  Port=2
  wires:
  seleccion/1 -> MATLAB Function/2(seleccion)
  m_est/1 -> MATLAB Function1/1(m_est)
  Delay One Step/1 -> MATLAB Function3/2(Thm_ref)
  yh_enc/1 -> MATLAB Function3/1(yh_enc)
  MATLAB Function3/1(vh_obs) -> MATLAB Function1/3(vh_obs), vh_obs/1
  vy_cmd/1 -> MATLAB Function/1(vy_cmd)
  MATLAB Function/1(vh_ref) -> MATLAB Function1/2(vh_ref)
  AND/1 -> MATLAB Function1/4(BRK)
  BRK_hE/1 -> AND/2
  vh_lim/1 -> MATLAB Function/3(vh_lim)
  BRK_h/1 -> AND/1
  MATLAB Function1/1(Thm_ref) -> Delay One Step/1, Thm_ref/1

== system modelo_planta_CODESYS_EXPERIMENTAL/Modulador Carro1 ==
  Ttm_ref : Inport
  BRK_t : Inport  Port=2
  Constant : Constant  Value=Ttm_Max
  Gain1 : Gain  Gain=-1
  Gain2 : Gain  Gain=1/tau_tm
  Integrator : Integrator  InitialCondition=Ttm_0
  Product : Product
  Saturation Dynamic : simulink/Discontinuities/Saturation Dynamic  OutMin=[]  OutMax=[]  OutDataTypeStr=Inherit: Same as second input  OutDataType=fixdt(1, 16)  OutScaling=2^-10  DoSatur=off
  Sum : Sum  Inputs=|+-
  Ttm : Outport
  wires:
  Constant/1 -> Saturation Dynamic/1, Gain1/1
  Gain1/1 -> Saturation Dynamic/3
  Saturation Dynamic/1 -> Sum/1  "Ttm_lim"
  Sum/1 -> Gain2/1
  Gain2/1 -> Integrator/1
  Integrator/1 -> Ttm/1, Sum/2
  Ttm_ref/1 -> Product/1
  BRK_t/1 -> Product/2
  Product/1 -> Saturation Dynamic/2

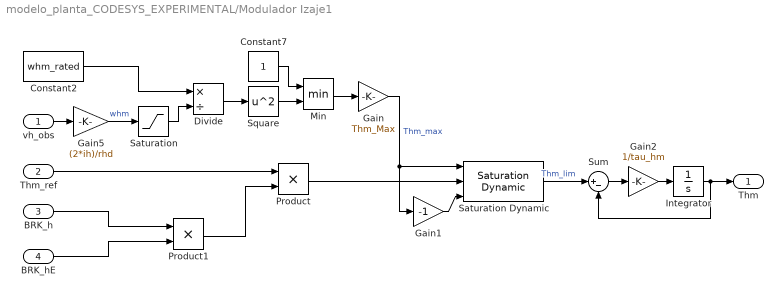
== system modelo_planta_CODESYS_EXPERIMENTAL/Modulador Izaje1 ==
  vh_obs : Inport
  Thm_ref : Inport  Port=2
  BRK_h : Inport  Port=3
  BRK_hE : Inport  Port=4
  Constant2 : Constant  Value=whm_rated
  Constant7 : Constant
  Divide : Product  Inputs=*/
  Gain : Gain  Gain=Thm_Max
  Gain1 : Gain  Gain=-1
  Gain2 : Gain  Gain=1/tau_hm
  Gain5 : Gain  Gain=(2*ih)/rhd
  Integrator : Integrator  InitialCondition=Thm_0
  Min : MinMax  Inputs=2
  Product : Product
  Product1 : Product
  Saturation : Saturate  UpperLimit=inf  LowerLimit=whm_rated
  Saturation Dynamic : simulink/Discontinuities/Saturation Dynamic  OutMin=[]  OutMax=[]  OutDataTypeStr=Inherit: Same as second input  OutDataType=fixdt(1, 16)  OutScaling=2^-10  DoSatur=off
  Square : Math  Operator=square
  Sum : Sum  Inputs=|+-
  Thm : Outport
  wires:
  Constant2/1 -> Divide/1
  Min/1 -> Gain/1
  Constant7/1 -> Min/1
  Gain/1 -> Gain1/1, Saturation Dynamic/1  "Thm_max"
  Saturation/1 -> Divide/2
  Square/1 -> Min/2
  Divide/1 -> Square/1
  vh_obs/1 -> Gain5/1
  Gain1/1 -> Saturation Dynamic/3
  Saturation Dynamic/1 -> Sum/1  "Thm_lim"
  Sum/1 -> Gain2/1
  Gain2/1 -> Integrator/1
  Integrator/1 -> Thm/1, Sum/2
  Thm_ref/1 -> Product/1
  BRK_h/1 -> Product1/1
  Product/1 -> Saturation Dynamic/2
  BRK_hE/1 -> Product1/2
  Product1/1 -> Product/2
  Gain5/1 -> Saturation/1  "whm"

== system modelo_planta_CODESYS_EXPERIMENTAL/Sensores Carro1 ==
  xt : Inport
  θtm : Inport  Port=2
  Encoder Carro : Subsystem
  Fines de carrera carro (rieles) : Subsystem
  xtd_enc : Outport
  FCE_izquierdo : Outport  Port=2
  FCE_derecho : Outport  Port=3
  FC_izquierdo : Outport  Port=4
  FC_derecho : Outport  Port=5
  wires:
  Fines de carrera carro (rieles)/1(FC_derecho) -> FC_derecho/1
  θtm/1 -> Encoder Carro/1(θtm)
  Fines de carrera carro (rieles)/2(FC_izquierdo) -> FC_izquierdo/1
  Fines de carrera carro (rieles)/3(FCE_derecho) -> FCE_derecho/1
  Fines de carrera carro (rieles)/4(FCE_izquierdo) -> FCE_izquierdo/1
  xt/1 -> Fines de carrera carro (rieles)/1(xt)
  Encoder Carro/1(xtd_enc) -> xtd_enc/1

== system modelo_planta_CODESYS_EXPERIMENTAL/Sensores Izaje1 ==
  θhm : Inport
  Encoder Izaje : Subsystem
  Fines de carrera izaje (tambor) : Subsystem
  yh_enc : Outport
  FCE_inferior : Outport  Port=2
  FCE_superior : Outport  Port=3
  FC_inferior : Outport  Port=4
  FC_superior : Outport  Port=5
  wires:
  Fines de carrera izaje (tambor)/1(FC_superior) -> FC_superior/1
  Fines de carrera izaje (tambor)/4(FCE_inferior) -> FCE_inferior/1
  Fines de carrera izaje (tambor)/2(FC_inferior) -> FC_inferior/1
  Encoder Izaje/1(yh_enc) -> Fines de carrera izaje (tambor)/1(y_enc), yh_enc/1
  θhm/1 -> Encoder Izaje/1(θhm)
  Fines de carrera izaje (tambor)/3(FCE_superior) -> FCE_superior/1

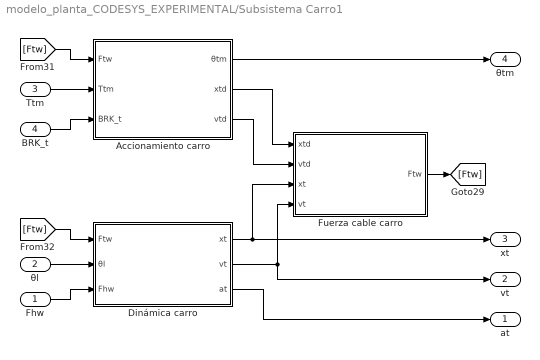
== system modelo_planta_CODESYS_EXPERIMENTAL/Subsistema Carro1 ==
  Fhw : Inport
  θl : Inport  Port=2
  Ttm : Inport  Port=3
  BRK_t : Inport  Port=4
  Accionamiento carro : Subsystem
  Dinámica carro : Subsystem
  Fuerza cable carro : Subsystem
  at : Outport
  vt : Outport  Port=2
  xt : Outport  Port=3
  θtm : Outport  Port=4
  wires:
  [Ftw] -> Accionamiento carro/1(Ftw)
  Accionamiento carro/1(θtm) -> θtm/1
  Dinámica carro/1(xt) -> Fuerza cable carro/3(xt), xt/1
  BRK_t/1 -> Accionamiento carro/3(BRK_t)
  [Ftw] -> Dinámica carro/1(Ftw)
  θl/1 -> Dinámica carro/2(θl)
  Ttm/1 -> Accionamiento carro/2(Ttm)
  Fuerza cable carro/1(Ftw) -> [Ftw]
  Dinámica carro/2(vt) -> Fuerza cable carro/4(vt), vt/1
  Accionamiento carro/2(xtd) -> Fuerza cable carro/1(xtd)
  Accionamiento carro/3(vtd) -> Fuerza cable carro/2(vtd)
  Fhw/1 -> Dinámica carro/3(Fhw)
  Dinámica carro/3(at) -> at/1

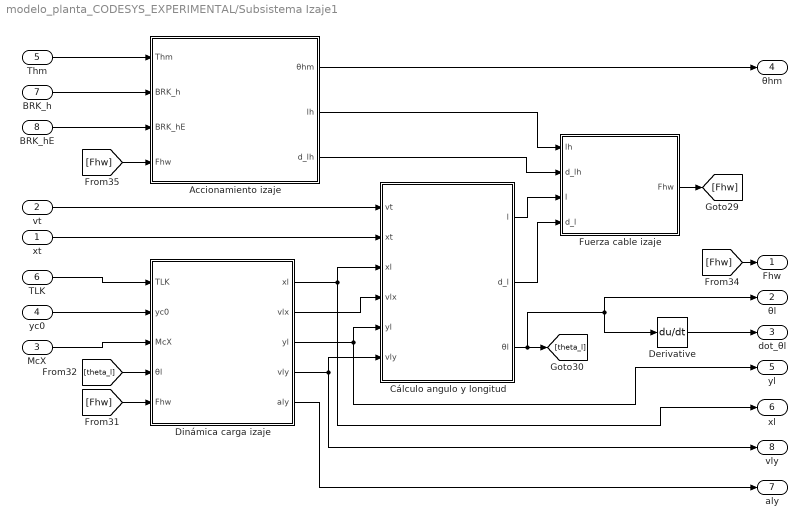
== system modelo_planta_CODESYS_EXPERIMENTAL/Subsistema Izaje1 ==
  xt : Inport
  vt : Inport  Port=2
  McX : Inport  Port=3
  yc0 : Inport  Port=4
  Thm : Inport  Port=5
  TLK : Inport  Port=6
  BRK_h : Inport  Port=7
  BRK_hE : Inport  Port=8
  Accionamiento izaje : Subsystem
  Cálculo angulo y longitud : Subsystem
  Derivative : Derivative
  Dinámica carga izaje : Subsystem
  Fuerza cable izaje : Subsystem
  Fhw : Outport
  θl : Outport  Port=2
  dot_θl : Outport  Port=3
  θhm : Outport  Port=4
  yl : Outport  Port=5
  xl : Outport  Port=6
  aly : Outport  Port=7
  vly : Outport  Port=8
  wires:
  vt/1 -> Cálculo angulo y longitud/1(vt)
  Accionamiento izaje/2(lh) -> Fuerza cable izaje/1(lh)
  yc0/1 -> Dinámica carga izaje/2(yc0)
  McX/1 -> Dinámica carga izaje/3(McX)
  Dinámica carga izaje/4(vly) -> vly/1, Cálculo angulo y longitud/6(vly)
  [Fhw] -> Accionamiento izaje/4(Fhw)
  [theta_l] -> Dinámica carga izaje/4(θl)
  xt/1 -> Cálculo angulo y longitud/2(xt)
  BRK_h/1 -> Accionamiento izaje/2(BRK_h)
  Dinámica carga izaje/1(xl) -> Cálculo angulo y longitud/3(xl), xl/1
  Dinámica carga izaje/2(vlx) -> Cálculo angulo y longitud/4(vlx)
  Fuerza cable izaje/1(Fhw) -> [Fhw]
  Cálculo angulo y longitud/1(l) -> Fuerza cable izaje/3(l)
  Accionamiento izaje/1(θhm) -> θhm/1
  Cálculo angulo y longitud/3(θl) -> θl/1, Derivative/1, [theta_l]
  TLK/1 -> Dinámica carga izaje/1(TLK)
  [Fhw] -> Dinámica carga izaje/5(Fhw)
  BRK_hE/1 -> Accionamiento izaje/3(BRK_hE)
  Thm/1 -> Accionamiento izaje/1(Thm)
  Dinámica carga izaje/3(yl) -> Cálculo angulo y longitud/5(yl), yl/1
  Cálculo angulo y longitud/2(d_l) -> Fuerza cable izaje/4(d_l)
  Accionamiento izaje/3(d_lh) -> Fuerza cable izaje/2(d_lh)
  Dinámica carga izaje/5(aly) -> aly/1
  [Fhw] -> Fhw/1
  Derivative/1 -> dot_θl/1

== system modelo_planta_CODESYS_EXPERIMENTAL/Sensores Carro1/Encoder Carro ==
  θtm : Inport
  Gain1 : Gain  Gain=rtd/it
  xtd_enc : Outport
  wires:
  θtm/1 -> Gain1/1
  Gain1/1 -> xtd_enc/1

== system modelo_planta_CODESYS_EXPERIMENTAL/Sensores Carro1/Fines de carrera carro (rieles) ==
  xt : Inport
  Compare To Constant : simulink/Logic and Bit Operations/Compare To Constant  relop=>=  const=xt_max  OutDataTypeStr=boolean
  Compare To Constant1 : simulink/Logic and Bit Operations/Compare To Constant  relop=>=  const=xt_max+0.5  OutDataTypeStr=boolean
  Compare To Constant2 : simulink/Logic and Bit Operations/Compare To Constant  relop=<=  const=xt_min  OutDataTypeStr=boolean
  Compare To Constant3 : simulink/Logic and Bit Operations/Compare To Constant  relop=<=  const=xt_min-0.5  OutDataTypeStr=boolean
  FC_derecho : Outport
  FC_izquierdo : Outport  Port=2
  FCE_derecho : Outport  Port=3
  FCE_izquierdo : Outport  Port=4
  wires:
  Compare To Constant2/1 -> FC_izquierdo/1
  xt/1 -> Compare To Constant/1, Compare To Constant1/1, Compare To Constant2/1, Compare To Constant3/1
  Compare To Constant3/1 -> FCE_izquierdo/1
  Compare To Constant1/1 -> FCE_derecho/1
  Compare To Constant/1 -> FC_derecho/1

== system modelo_planta_CODESYS_EXPERIMENTAL/Sensores Izaje1/Encoder Izaje ==
  θhm : Inport
  Gain3 : Gain  Gain=rhd/(2*ih)
  yh_enc : Outport
  wires:
  θhm/1 -> Gain3/1
  Gain3/1 -> yh_enc/1

== system modelo_planta_CODESYS_EXPERIMENTAL/Sensores Izaje1/Fines de carrera izaje (tambor) ==
  y_enc : Inport
  Compare To Constant4 : simulink/Logic and Bit Operations/Compare To Constant  relop=>=  const=yh_max  OutDataTypeStr=boolean
  Compare To Constant5 : simulink/Logic and Bit Operations/Compare To Constant  relop=>=  const=yh_max+0.5  OutDataTypeStr=boolean
  Compare To Constant6 : simulink/Logic and Bit Operations/Compare To Constant  relop=<=  const=yh_min  OutDataTypeStr=boolean
  Compare To Constant7 : simulink/Logic and Bit Operations/Compare To Constant  relop=<=  const=yh_min-0.5  OutDataTypeStr=boolean
  FC_superior : Outport
  FC_inferior : Outport  Port=2
  FCE_superior : Outport  Port=3
  FCE_inferior : Outport  Port=4
  wires:
  Compare To Constant7/1 -> FCE_inferior/1
  y_enc/1 -> Compare To Constant7/1, Compare To Constant6/1, Compare To Constant4/1, Compare To Constant5/1
  Compare To Constant6/1 -> FC_inferior/1
  Compare To Constant5/1 -> FCE_superior/1
  Compare To Constant4/1 -> FC_superior/1

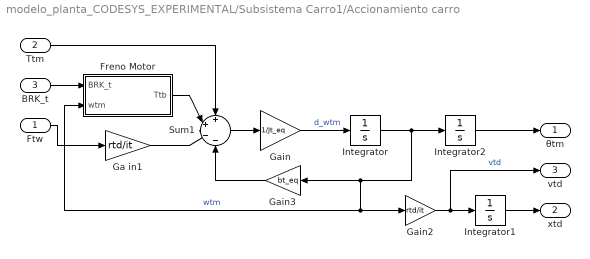
== system modelo_planta_CODESYS_EXPERIMENTAL/Subsistema Carro1/Accionamiento carro ==
  Ftw : Inport
  Ttm : Inport  Port=2
  BRK_t : Inport  Port=3
  Freno Motor : Subsystem
  Ga in1 : Gain  Gain=rtd/it
  Gain : Gain  Gain=1/Jt_eq
  Gain2 : Gain  Gain=rtd/it
  Gain3 : Gain  Gain=bt_eq
  Integrator : Integrator  InitialCondition=wtm_0
  Integrator1 : Integrator  InitialCondition=xtd_0
  Integrator2 : Integrator  InitialCondition=titatm_0
  Sum1 : Sum  Inputs=++--
  θtm : Outport
  xtd : Outport  Port=2
  vtd : Outport  Port=3
  wires:
  Sum1/1 -> Gain/1
  Integrator/1 -> Gain2/1, Freno Motor/2(wtm), Gain3/1, Integrator2/1  "wtm"
  Gain2/1 -> Integrator1/1, vtd/1  "vtd"
  Ttm/1 -> Sum1/1
  Gain/1 -> Integrator/1  "d_wtm"
  BRK_t/1 -> Freno Motor/1(BRK_t)
  Integrator1/1 -> xtd/1
  Ftw/1 -> Ga in1/1
  Ga in1/1 -> Sum1/3
  Freno Motor/1(Ttb) -> Sum1/2
  Gain3/1 -> Sum1/4
  Integrator2/1 -> θtm/1

== system modelo_planta_CODESYS_EXPERIMENTAL/Subsistema Carro1/Dinámica carro ==
  Ftw : Inport
  θl : Inport  Port=2
  Fhw : Inport  Port=3
  Gain : Gain  Gain=2
  Gain1 : Gain  Gain=1/Mt
  Gain2 : Gain  Gain=bt
  Integrator : Integrator  InitialCondition=vt_0
  Integrator1 : Integrator  InitialCondition=xt_0
  Product : Product
  Sin : Trigonometry
  Sum : Sum  Inputs=++-
  xt : Outport
  vt : Outport  Port=2
  at : Outport  Port=3
  wires:
  Gain1/1 -> at/1, Integrator/1  "dot_vt"
  Integrator/1 -> Gain2/1, vt/1, Integrator1/1  "vt"
  Gain2/1 -> Sum/3
  Sum/1 -> Gain1/1
  Integrator1/1 -> xt/1  "xt"
  Fhw/1 -> Gain/1
  Gain/1 -> Product/2
  θl/1 -> Sin/1
  Sin/1 -> Product/1
  Product/1 -> Sum/2  "F_coupling"
  Ftw/1 -> Sum/1

== system modelo_planta_CODESYS_EXPERIMENTAL/Subsistema Carro1/Fuerza cable carro ==
  xtd : Inport
  vtd : Inport  Port=2
  xt : Inport  Port=3
  vt : Inport  Port=4
  Gain : Gain  Gain=Ktw
  Gain1 : Gain  Gain=btw
  Sum : Sum  Inputs=+-
  Sum1 : Sum
  Sum2 : Sum  Inputs=+-
  Ftw : Outport
  wires:
  xtd/1 -> Sum/1
  Gain1/1 -> Sum1/2
  Sum/1 -> Gain/1
  xt/1 -> Sum/2
  Sum2/1 -> Gain1/1
  Gain/1 -> Sum1/1
  vt/1 -> Sum2/2
  Sum1/1 -> Ftw/1  "Ftw"
  vtd/1 -> Sum2/1

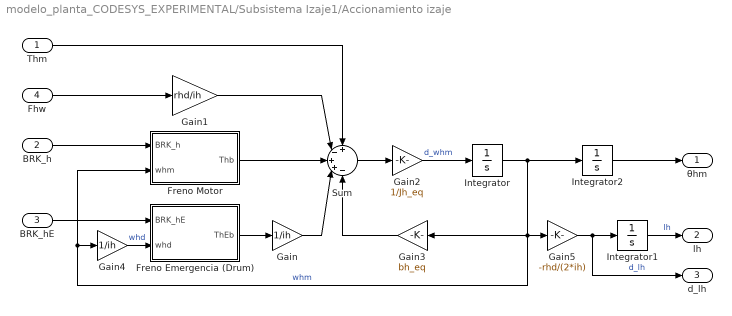
== system modelo_planta_CODESYS_EXPERIMENTAL/Subsistema Izaje1/Accionamiento izaje ==
  Thm : Inport
  BRK_h : Inport  Port=2
  BRK_hE : Inport  Port=3
  Fhw : Inport  Port=4
  Freno Emergencia (Drum) : Subsystem
  Freno Motor : Subsystem
  Gain : Gain  Gain=1/ih
  Gain1 : Gain  Gain=rhd/ih
  Gain2 : Gain  Gain=1/Jh_eq
  Gain3 : Gain  Gain=bh_eq
  Gain4 : Gain  Gain=1/ih
  Gain5 : Gain  Gain=-rhd/(2*ih)
  Integrator : Integrator  InitialCondition=whm_0
  Integrator1 : Integrator  InitialCondition=lh_0
  Integrator2 : Integrator  InitialCondition=titahm_0
  Sum : Sum  Inputs=+-++-
  θhm : Outport
  lh : Outport  Port=2
  d_lh : Outport  Port=3
  wires:
  Gain5/1 -> d_lh/1, Integrator1/1  "d_lh"
  Integrator/1 -> Gain3/1, Freno Motor/2(whm), Gain4/1, Gain5/1, Integrator2/1  "whm"
  Freno Emergencia (Drum)/1(ThEb) -> Gain/1
  Gain3/1 -> Sum/5
  BRK_h/1 -> Freno Motor/1(BRK_h)
  Gain/1 -> Sum/4
  Gain2/1 -> Integrator/1  "d_whm"
  Sum/1 -> Gain2/1
  Gain4/1 -> Freno Emergencia (Drum)/2(whd)  "whd"
  BRK_hE/1 -> Freno Emergencia (Drum)/1(BRK_hE)
  Fhw/1 -> Gain1/1
  Freno Motor/1(Thb) -> Sum/3
  Gain1/1 -> Sum/2
  Integrator1/1 -> lh/1  "lh"
  Integrator2/1 -> θhm/1
  Thm/1 -> Sum/1

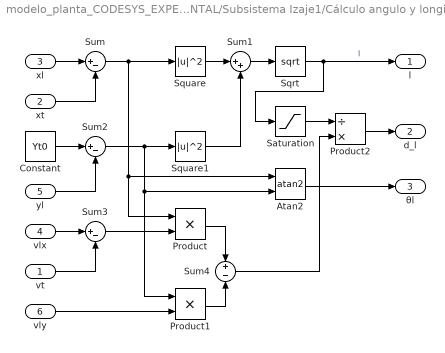
== system modelo_planta_CODESYS_EXPERIMENTAL/Subsistema Izaje1/Cálculo angulo y longitud ==
  vt : Inport
  xt : Inport  Port=2
  xl : Inport  Port=3
  vlx : Inport  Port=4
  yl : Inport  Port=5
  vly : Inport  Port=6
  Atan2 : Trigonometry  Operator=atan2
  Constant : Constant  Value=Yt0
  Product : Product
  Product1 : Product
  Product2 : Product  Inputs=/*
  Saturation : Saturate  UpperLimit=inf  LowerLimit=0.1
  Sqrt : Sqrt
  Square : Math  Operator=magnitude^2
  Square1 : Math  Operator=magnitude^2
  Sum : Sum  Inputs=|+-
  Sum1 : Sum  Inputs=|++
  Sum2 : Sum  Inputs=|+-
  Sum3 : Sum  Inputs=|+-
  Sum4 : Sum  Inputs=+-
  l : Outport
  d_l : Outport  Port=2
  θl : Outport  Port=3
  wires:
  Product2/1 -> d_l/1
  Sqrt/1 -> l/1, Saturation/1  "l"
  Sum1/1 -> Sqrt/1
  Sum2/1 -> Product1/1, Atan2/2, Square1/1
  Sum/1 -> Product/1, Atan2/1, Square/1
  yl/1 -> Sum2/2
  Atan2/1 -> θl/1
  vly/1 -> Product1/2
  xl/1 -> Sum/1
  Constant/1 -> Sum2/1
  Sum3/1 -> Product/2
  Square1/1 -> Sum1/2
  vt/1 -> Sum3/2
  Sum4/1 -> Product2/2
  vlx/1 -> Sum3/1
  xt/1 -> Sum/2
  Square/1 -> Sum1/1
  Product1/1 -> Sum4/2
  Product/1 -> Sum4/1
  Saturation/1 -> Product2/1
